simulink model "button_to_pwm"  (R2017a)
settings: Solver=FixedStepDiscrete  StartTime=0.0  StopTime=50000  FixedStep=1  RelTol=1e-3
libraries: hdlsllib x4, simulink x3
settings Model: Creator=chandler.ga  LastModifiedBy=chandler.ga

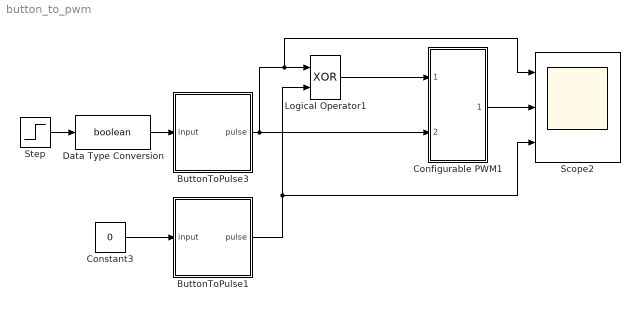
== system button_to_pwm ==
  ButtonToPulse1 : Subsystem
  ButtonToPulse3 : Subsystem
  Configurable PWM1 : Subsystem
  Constant3 : Constant  Value=0  OutDataTypeStr=boolean
  Data Type Conversion : DataTypeConversion  OutDataTypeStr=boolean
  Logical Operator1 : Logic  Operator=XOR  IconShape=distinctive  AllPortsSameDT=off  OutDataTypeStr=boolean
  Scope2 : Scope  NumInputPorts=3
  Step : Step  Time=25000  Before=1  After=0  SampleTime=0
  wires:
  Logical Operator1/1 -> Configurable PWM1/1(Enable)
  ButtonToPulse1/1(pulse) -> Scope2/3, Logical Operator1/2
  ButtonToPulse3/1(pulse) -> Configurable PWM1/2(Direction), Scope2/1, Logical Operator1/1
  Configurable PWM1/1(PWM) -> Scope2/2
  Step/1 -> Data Type Conversion/1
  Constant3/1 -> ButtonToPulse1/1(input)
  Data Type Conversion/1 -> ButtonToPulse3/1(input)

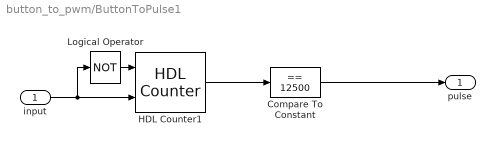
== system button_to_pwm/ButtonToPulse1 ==
  input : Inport
  Compare To Constant : simulink/Logic and Bit Operations/Compare To Constant  relop===  const=12500  OutDataTypeStr=boolean
  HDL Counter1 : hdlsllib/HDL Operations/HDL Counter  CountType=Count limited  CountInit=0  CountStep=1  CountMax=50000  CountFromType=Initial value  CountFrom=0  CountResetPort=on  CountLoadPort=off  CountEnbPort=on  CountDirPort=off  CountDataType=Unsigned  CountWordLen=18  CountFracLen=0  CountSampTime=1
      settings: SourceProductName=HDL Coder  SourceProductBaseCode=HD
  Logical Operator : Logic  Operator=NOT  IconShape=distinctive  AllPortsSameDT=off  OutDataTypeStr=boolean
  pulse : Outport
  wires:
  HDL Counter1/1 -> Compare To Constant/1
  input/1 -> Logical Operator/1, HDL Counter1/2
  Compare To Constant/1 -> pulse/1
  Logical Operator/1 -> HDL Counter1/1

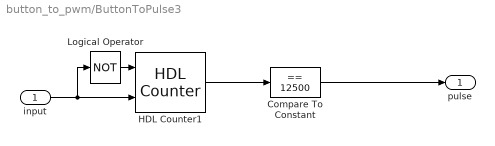
== system button_to_pwm/ButtonToPulse3 ==
  input : Inport
  Compare To Constant : simulink/Logic and Bit Operations/Compare To Constant  relop===  const=12500  OutDataTypeStr=boolean
  HDL Counter1 : hdlsllib/HDL Operations/HDL Counter  CountType=Count limited  CountInit=0  CountStep=1  CountMax=50000  CountFromType=Initial value  CountFrom=0  CountResetPort=on  CountLoadPort=off  CountEnbPort=on  CountDirPort=off  CountDataType=Unsigned  CountWordLen=18  CountFracLen=0  CountSampTime=1
      settings: SourceProductName=HDL Coder  SourceProductBaseCode=HD
  Logical Operator : Logic  Operator=NOT  IconShape=distinctive  AllPortsSameDT=off  OutDataTypeStr=boolean
  pulse : Outport
  wires:
  HDL Counter1/1 -> Compare To Constant/1
  input/1 -> Logical Operator/1, HDL Counter1/2
  Compare To Constant/1 -> pulse/1
  Logical Operator/1 -> HDL Counter1/1

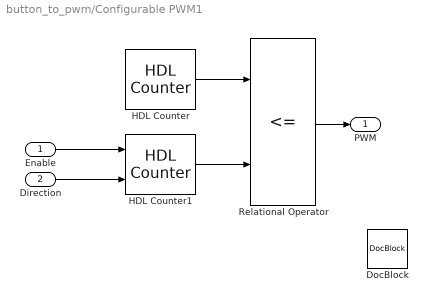
== system button_to_pwm/Configurable PWM1 ==
  Enable : Inport
  Direction : Inport  Port=2
  DocBlock : simulink/Model-Wide Utilities/DocBlock  DocumentType=Text
      content=|
      | First pulse is 76 thangs (1.2012*10^4 and 1.2088*10^4) and the other is 82 (1.3013*10^4 and 1.3095*10^4)
  HDL Counter : hdlsllib/HDL Operations/HDL Counter  CountType=Count limited  CountInit=0  CountStep=1  CountMax=1000  CountFromType=Initial value  CountFrom=0  CountResetPort=off  CountLoadPort=off  CountEnbPort=off  CountDirPort=off  CountDataType=Unsigned  CountWordLen=10  CountFracLen=0  CountSampTime=1
      settings: SourceProductName=HDL Coder  SourceProductBaseCode=HD
  HDL Counter1 : hdlsllib/HDL Operations/HDL Counter  CountType=Count limited  CountInit=75  CountStep=6  CountMax=120  CountFromType=Specify  CountFrom=30  CountResetPort=off  CountLoadPort=off  CountEnbPort=on  CountDirPort=on  CountDataType=Unsigned  CountWordLen=7  CountFracLen=0  CountSampTime=1
      settings: SourceProductName=HDL Coder  SourceProductBaseCode=HD
  Relational Operator : RelationalOperator  Operator=<=  OutDataTypeStr=boolean  RndMeth=Simplest
  PWM : Outport
  wires:
  Direction/1 -> HDL Counter1/2
  Relational Operator/1 -> PWM/1
  Enable/1 -> HDL Counter1/1
  HDL Counter1/1 -> Relational Operator/2
  HDL Counter/1 -> Relational Operator/1
